simulink model "Ex_4"  (Simulink 8.0)
settings: Solver=ode45  StartTime=0.0  StopTime=10.0  RelTol=1e-3
settings Model: Creator=Faradars  LastModifiedBy=Faradars

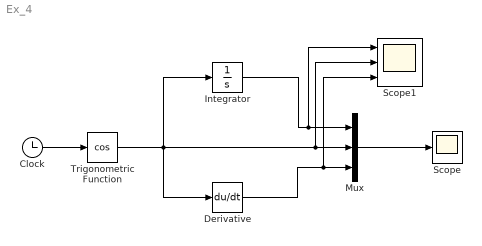
== system Ex_4 ==
  Clock : Clock
  Derivative : Derivative
  Integrator : Integrator
  Mux : Mux  Inputs=3
  Scope : Scope
  Scope1 : Scope  NumInputPorts=3
      settings: YMin=-5~-5~-5  YMax=5~5~5
  Trigonometric Function : Trigonometry  Operator=cos
  wires:
  Clock/1 -> Trigonometric Function/1
  Trigonometric Function/1 -> Scope1/2, Mux/2, Derivative/1, Integrator/1
  Integrator/1 -> Scope1/1, Mux/1
  Derivative/1 -> Scope1/3, Mux/3
  Mux/1 -> Scope/1
